simulink model "linea2"  (Simulink 4.00)
settings: Solver=ode45  StartTime=0.0  StopTime=10.0  RelTol=1e-3
settings Model: LastModifiedBy=Administrator  BlockReductionOpt=off

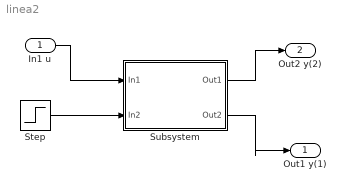
== system linea2 ==
  In1 u : Inport  Port=1
  Step : Step  Time=1  Before=0  After=1  SampleTime=0
  Subsystem : Subsystem
      settings: RTWFcnNameOpts=Auto  RTWFileNameOpts=Auto
  Out1 y(1) : Outport  Port=1
  Out2 y(2) : Outport  Port=2
  wires:
  Step/1 -> Subsystem/2(In2)
  In1 u/1 -> Subsystem/1(In1)
  Subsystem/1(Out1) -> Out2 y(2)/1
  Subsystem/2(Out2) -> Out1 y(1)/1

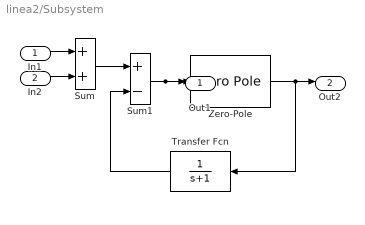
== system linea2/Subsystem ==
  In1 : Inport  Port=1
  In2 : Inport  Port=2
  Sum : Sum  Inputs=++  SaturateOnIntegerOverflow=on
  Sum1 : Sum  Inputs=+-  SaturateOnIntegerOverflow=on
  Transfer Fcn : TransferFcn  Orientation=left  Numerator=[1]  Denominator=[1 1]  Realization=auto  AbsoluteTolerance=auto
  Zero-Pole : ZeroPole  Zeros=[-0.6]  Poles=[0 -0.5]  Gain=[0.1]  AbsoluteTolerance=auto
  Out1 : Outport  Port=1
  Out2 : Outport  Port=2
  wires:
  Sum/1 -> Sum1/1
  Sum1/1 -> Zero-Pole/1, Out1/1
  Transfer Fcn/1 -> Sum1/2
  Zero-Pole/1 -> Transfer Fcn/1, Out2/1
  In1/1 -> Sum/1
  In2/1 -> Sum/2
